simulink model "LQRFirstClosedLoopOld"  (R2018b)
settings: Solver=VariableStepAuto  StartTime=0.0  StopTime=10.0  RelTol=1e-3
values from neighbouring files (symbols this model uses):
  A = [0 0 1 0; 0 0 0 1; 0 -m*g/Mc -Kg^2*Km*Kb/(Mc*Rm*r^2) 0; 0 (Mc+m)*g/(Mc*l) Kg^2*Km*Kb/(Mc*Rm*r^2*l) 0]    [INVERTEDPENDULUM.m]    (also in InvertedPendulum.m)
  B = [0; 0; Km*Kg/(Mc*Rm*r); -Km*Kg/(r*Rm*Mc*l)]    [INVERTEDPENDULUM.m]    (also in InvertedPendulum.m)
  C = eye(4,4)    [INVERTEDPENDULUM.m]    (also in InvertedPendulum.m)
  D = zeros(4,1)    [INVERTEDPENDULUM.m]    (also in InvertedPendulum.m)
  intial_State = [0;0;0;0]    [INVERTEDPENDULUM.m]    (also in InvertedPendulum.m)
  K = lqr(system_open,Q,R)    [INVERTEDPENDULUM.m]    (also in InvertedPendulum.m)
  reference_State = [1;0;0;0]    [INVERTEDPENDULUM.m]    (also in InvertedPendulum.m = [0;0;0;0])
settings Model: Creator=jan  LastModifiedBy=jan

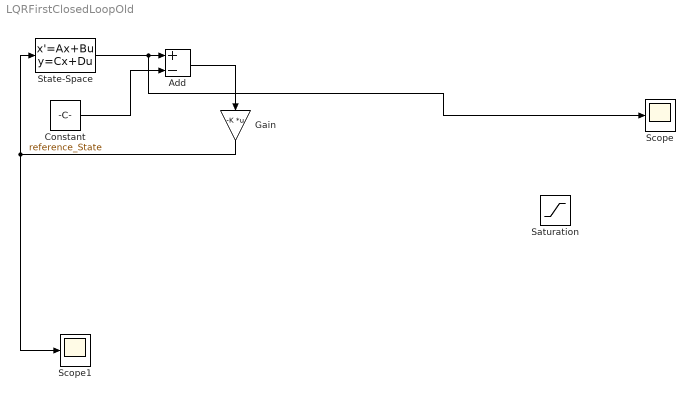
== system LQRFirstClosedLoopOld ==
  Add : Sum  Inputs=+-
  Constant : Constant  Value=reference_State
  Gain : Gain  Gain=-K  Multiplication=Matrix(K*u) (u vector)
  Saturation : Saturate  UpperLimit=10  LowerLimit=-10
  Scope : Scope
  Scope1 : Scope
  State-Space : StateSpace  A=A  B=B  C=C  D=D  InitialCondition=intial_State
  wires:
  Constant/1 -> Add/2
  State-Space/1 -> Scope/1, Add/1
  Add/1 -> Gain/1
  Gain/1 -> State-Space/1, Scope1/1
